simulink model "Control_Block_Diagram"  (R2018b)
settings: Solver=VariableStepAuto  StartTime=0.0  StopTime=100  RelTol=1e-3
settings Model: Creator=sdozi  LastModifiedBy=sdozi

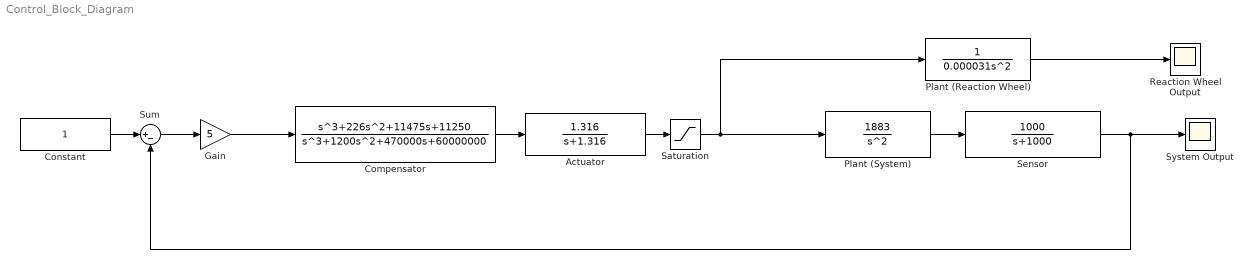
== system Control_Block_Diagram ==
  Actuator : TransferFcn  Numerator=[1.316]  Denominator=[1 1.316]
  Compensator : TransferFcn  Numerator=[1 226 11475 11250]  Denominator=[1 1200 470000 60000000]
  Constant : Constant
  "Gain " : Gain  Gain=5
  Plant (Reaction Wheel) : TransferFcn  Denominator=[0.000031 0 0]
  Plant (System) : TransferFcn  Numerator=[1883]  Denominator=[1 0 0]
  Reaction Wheel Output : Scope
  Saturation : Saturate  UpperLimit=0.007  LowerLimit=-0.007
  Sensor : TransferFcn  Numerator=[1000]  Denominator=[1 1000]
  Sum : Sum  Inputs=|+-
  System Output : Scope
  wires:
  Constant/1 -> Sum/1
  Sum/1 -> "Gain "/1
  Plant (Reaction Wheel)/1 -> Reaction Wheel Output/1
  Plant (System)/1 -> Sensor/1
  Actuator/1 -> Saturation/1
  Sensor/1 -> Sum/2, System Output/1
  Compensator/1 -> Actuator/1
  Saturation/1 -> Plant (System)/1, Plant (Reaction Wheel)/1
  "Gain "/1 -> Compensator/1
